simulink model "HDVPSG_DelayComp_NewRef_RealDrop_case1"  (R2019b)
settings: Solver=FixedStepDiscrete  StartTime=0.0  StopTime=28  FixedStep=UT.Ts_Veh  RelTol=1e-3
PostLoadFcn:
  | if any(exist('dsrtsu_mdlpostloadfcn', 'file') ~= 0), dsrtsu_mdlpostloadfcn('Execute', bdroot); end
InitFcn:
  | , if any(exist('dsmpb_private', 'file') ~= 0), dsmpb_private('dsmpb_mdlclblib', 'Init', bdroot); end,
values from neighbouring files (symbols this model uses):
  BETA_HDV_Leader = 50    [HDVPSG_DelayComp_NewRef_RealDrop_script_case1.m]
  BETA_PSG_Follower = 150    [HDVPSG_DelayComp_NewRef_RealDrop_script_case1.m]
  CtrlZone_Length = 250    [HDVPSG_DelayComp_NewRef_RealDrop_script_case1.m]
  DELTA_D_MIN = 5    [HDVPSG_DelayComp_NewRef_RealDrop_script_case1.m]
  DELTA_DR_MG_TCC = 15    [HDVPSG_DelayComp_NewRef_RealDrop_script_case1.m]
  HDV_AMAX = 1.3    [HDVPSG_DelayComp_NewRef_RealDrop_script_case1.m]
  HDV_AMIN = -2.5    [HDVPSG_DelayComp_NewRef_RealDrop_script_case1.m]
  HDV_first_v0 = 13    [HDVPSG_DelayComp_NewRef_RealDrop_script_case1.m]
  HDV_HighMu_D = 9    [HDVPSG_DelayComp_NewRef_RealDrop_script_case1.m]
  HDV_HighMu_I = 27    [HDVPSG_DelayComp_NewRef_RealDrop_script_case1.m]
  HDV_HighMu_P = 27    [HDVPSG_DelayComp_NewRef_RealDrop_script_case1.m]
  HDV_HighMu_TRFC = 0.7    [HDVPSG_DelayComp_NewRef_RealDrop_script_case1.m]
  HDV_last_v0 = 13    [HDVPSG_DelayComp_NewRef_RealDrop_script_case1.m]
  HDV_LowMu_D = 6    [HDVPSG_DelayComp_NewRef_RealDrop_script_case1.m]
  HDV_LowMu_I = 8    [HDVPSG_DelayComp_NewRef_RealDrop_script_case1.m]
  HDV_LowMu_P = 12    [HDVPSG_DelayComp_NewRef_RealDrop_script_case1.m]
  HDV_LowMu_TRFC = 0.6    [HDVPSG_DelayComp_NewRef_RealDrop_script_case1.m]
  Np_MPC = 20    [HDVPSG_DelayComp_NewRef_RealDrop_script_case1.m]
  PSG_AMAX = 3.2    [HDVPSG_DelayComp_NewRef_RealDrop_script_case1.m]
  PSG_AMIN = -6    [HDVPSG_DelayComp_NewRef_RealDrop_script_case1.m]
  PSG_end_v0 = 13    [HDVPSG_DelayComp_NewRef_RealDrop_script_case1.m]
  PSG_first_v0 = 13    [HDVPSG_DelayComp_NewRef_RealDrop_script_case1.m]
  PSG_HighMu_D = 15    [HDVPSG_DelayComp_NewRef_RealDrop_script_case1.m]
  PSG_HighMu_I = 125    [HDVPSG_DelayComp_NewRef_RealDrop_script_case1.m]
  PSG_HighMu_P = 75    [HDVPSG_DelayComp_NewRef_RealDrop_script_case1.m]
  PSG_HighMu_TRFC = 0.8    [HDVPSG_DelayComp_NewRef_RealDrop_script_case1.m]
  PSG_LowMu_D = 12    [HDVPSG_DelayComp_NewRef_RealDrop_script_case1.m]
  PSG_LowMu_I = 64    [HDVPSG_DelayComp_NewRef_RealDrop_script_case1.m]
  PSG_LowMu_P = 48    [HDVPSG_DelayComp_NewRef_RealDrop_script_case1.m]
  PSG_LowMu_TRFC = 0.7    [HDVPSG_DelayComp_NewRef_RealDrop_script_case1.m]
  PSG_middle_v0 = 13    [HDVPSG_DelayComp_NewRef_RealDrop_script_case1.m]
  Q_Leader = 1    [HDVPSG_DelayComp_NewRef_RealDrop_script_case1.m]
  Qd_dot_PSG_Follower = 2    [HDVPSG_DelayComp_NewRef_RealDrop_script_case1.m]
  Qd_PSG_Follower = 10    [HDVPSG_DelayComp_NewRef_RealDrop_script_case1.m]
  R_Leader = 20    [HDVPSG_DelayComp_NewRef_RealDrop_script_case1.m]
  R_PSG_Follower = 1    [HDVPSG_DelayComp_NewRef_RealDrop_script_case1.m]
  Recved_40_1 = Recved_Flag_Combined(47740,:)    [HDVPSG_DelayComp_NewRef_RealDrop_script_case1.m]
  Recved_40_2 = Recved_Flag_Combined(47780,:)    [HDVPSG_DelayComp_NewRef_RealDrop_script_case1.m]
  Recved_40_3 = Recved_Flag_Combined(49536,:)    [HDVPSG_DelayComp_NewRef_RealDrop_script_case1.m]
  Recved_40_4 = Recved_Flag_Combined(118106,:)    [HDVPSG_DelayComp_NewRef_RealDrop_script_case1.m]
  Rho_deltad_PSG_Follower = 1e3    (= 1000)    [HDVPSG_DelayComp_NewRef_RealDrop_script_case1.m]
  Rho_v_PSG_Follower = 1e3    (= 1000)    [HDVPSG_DelayComp_NewRef_RealDrop_script_case1.m]
  T_ADE = 0.01    [HDVPSG_DelayComp_NewRef_RealDrop_script_case1.m]
  V_MAX = 40    [HDVPSG_DelayComp_NewRef_RealDrop_script_case1.m]
  V_MIN = 0    [HDVPSG_DelayComp_NewRef_RealDrop_script_case1.m]
  VR_MG_TCC = 15    [HDVPSG_DelayComp_NewRef_RealDrop_script_case1.m]
undefined symbols (not defined in the file or in its folder): DiscIntNeverNeededParam, UT
libraries: simulink x46
(part 3 of 16)

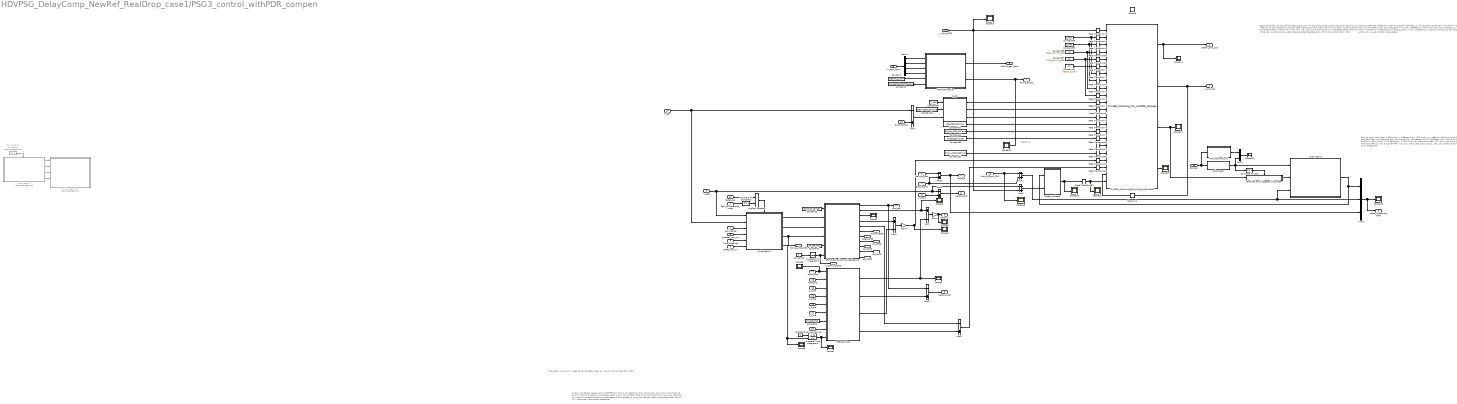
== system HDVPSG_DelayComp_NewRef_RealDrop_case1/PSG3_control_withPDR_compen ==
  note: As the immediate leader cannot PERFECTLY follow its reference, then there may be minor initial tracking errors in terms of delta_d and delta_d_dot, which can trigger large initial command
      |
      | One way to overcome this issue is to recalculate the parameters of the leader by using the leader's real-time states data. But it will introduce inconsistant reference
  note: For the case when Recv's frequency is different from MPC, then you need to make sure that the predicted step matches the real world time. So, we create a novel Lost-step block
      |
      | The commented one only works when V2VC freqeucny = MPC
      |
      | The max prediction step is 21, so if you have Large Sampling Period with a higher PDR, you may have step lost over 21. We just use the last one to fulfill the others.
  note: Adaptive
  note: Because Hc =1, so the diff of delta_d_dot_pre will equal the delta_ddot_hat as the MPC input.
      | That means, we cannot get the next Np step delta_ddot from MPC's solution; so the a of front car needs to be estimated in other ways.
      | For now, we just hold a_front once it is lost
      |
      | Because of a_front's influence, we cannot have accurate predicted delta_d_dot within the horizon from MPC
  note: Use the predicted states from MPC to replace lost delta_d, the results is quitewell;
      |
      | However, it does not work for delta_d_dot, the prediciton of d_dot is affected by both your command (delta_v_r), but more importantly, it depends on delta_d_ddot, which is affected by a_front. Unless you can predict a_front, or you cannot do it accurately.
  note: The green inputs only need to be inputted once. So, we do not consider their PDR.
  Ego_CtrL_enabled_Index : Inport
  t_all_leader : Inport  Port=2
  t_leader_has_run : Inport  Port=3
  t_PRE_has_run : Inport  Port=4
  Time_headway : Inport  Port=5
  Front_to_end : Inport  Port=6
  Ego_to_end : Inport  Port=7
  v_Front : Inport  Port=8
  v_Ego : Inport  Port=9
  a_Ego : Inport  Port=10
  XY_ego_front : Inport  Port=11
  Reset_sig : Inport  Port=12
  Front_to_end_PDR : Inport  Port=13
  v_Front_PDR : Inport  Port=14
  a_Front_PDR : Inport  Port=15
  Recved : Inport  Port=16
  alpha_pre : Inport  Port=17
  beta_pre : Inport  Port=18
  c_1_pre : Inport  Port=19
  c_2_pre : Inport  Port=20
  c_3_pre : Inport  Port=21
  c_4_pre : Inport  Port=22
  T_all_to_MP_pre : Inport  Port=23
  Enable : EnablePort
  Add : Sum  Inputs=+-
  Add{1..3,5..8} (7 alike) : Sum  Inputs=-+
  Add4 : Sum  Inputs=+-
  CVXGEN_Following_Car_Dist_Ctrl_NonSoft2 : S-Function  Description=Simulink:masks:SFunctionBuilder_MD  InitFcn=try, set_param(gcb,'FunctionName','CVXGEN_Following_Car_withPDR_Compen'), end  FunctionName=CVXGEN_Following_Car_withPDR_Compen  SFunctionModules=CVXGEN_Following_Car_withPDR_Compen_wrapper solver util matrix_support ldl  SFunctionDeploymentMode=off  EnableBusSupport=off
      mask init: same as HDVPSG_DelayComp_NewRef_RealDrop_case1/HDV2_control_withPDR_compen/CVXGEN_Following_Car_Dist_Ctrl_NonSoft2
      settings: CopyFcn=set_param(gcbh,'LinkStatus','none')  PreSaveFcn=try, set_param(gcb,'FunctionName','CVXGEN_Following_Car_withPDR_Compen'), end  OpenFcn=sfunctionwizard(gcbh)
      mask Display: plot(val(:,1),val(:,2)),disp(sys), port_label('input',1,'v_front_car'), port_label('input',2,'vmax'), port_label('input',3,'vmin'), port_label('input',4,'deltav_max'), port_label('input',5,'deltav_min'), port_label('input',6,'deltad_min'), port_label('input',7,'vcmd_max'), port_label('input',8,'vcmd_min'), port_label('input',9,'delta_vcmd_max'), port_label('input',10,'delta_vcmd_min'), port_label('input',11,'A'), port_label('input',12,'B'), port_label('input',13,'d_k'), port_label('input',14,'Q_deltad'), port_label('input',15,'Q_deltad_dot'), port_label('input',16,'R'), port_label('input',17,'Rho_deltad'), port_label('input',18,'Rho_v'), port_label('input',19,'deltad_r'), port_label('input',20,'deltad_dot_r'), port_label('input',21,'v_cmd_last'), port_label('input',22,'x_0'), port_label('output',1,'delta_v_cmd_opt'), port_label('output',2,'v_cmd_opt'), port_label('output',3,'delta_d_pre'), port_label('output',4,'delta_d_dot_pre')
  Compare To Constant2 : simulink/Logic and Bit Operations/Compare To Constant  relop===  const=1  OutDataTypeStr=boolean
  Compare To Constant3 : simulink/Logic and Bit Operations/Compare To Constant  Commented=on  relop===  const=1  OutDataTypeStr=boolean
  Compare To Zero : simulink/Logic and Bit Operations/Compare To Zero  relop===  OutDataTypeStr=boolean
  Constant : Constant  Value=DELTA_D_MIN
  Constant2 : Constant  Value=Rho_deltad_PSG_Follower
  Constant3 : Constant
  Constant4 : Constant  Value=VR_MG_TCC
  Constant42 : Constant  Value=T_ADE
  Constant43 : Constant  Value=Qd_PSG_Follower
  Constant44 : Constant  Value=Qd_dot_PSG_Follower
  Constant45 : Constant  Value=DELTA_D_MIN
  Constant5 : Constant
  Constant50 : Constant  Value=R_PSG_Follower
  Constant51 : Constant  Value=Rho_v_PSG_Follower
  Constant55 : Constant  Value=PSG_AMAX*T_ADE
  Constant57 : Constant  Value=PSG_AMIN*T_ADE
  Constant58 : Constant  Value=V_MAX
  Constant59 : Constant  Value=V_MIN
  Constant6 : Constant  Value=CtrlZone_Length
  Constant61 : Constant  Value=BETA_PSG_Follower
  Constant7 : Constant  Value=VR_MG_TCC
  Demux : Demux
  Discrete-Time Integrator1 : DiscreteIntegrator  SampleTime=-1  ICPrevOutput=DiscIntNeverNeededParam  ICPrevScaledInput=DiscIntNeverNeededParam
  Discrete-Time Integrator2 : DiscreteIntegrator  InitialConditionSource=external  SampleTime=-1  ICPrevOutput=DiscIntNeverNeededParam  ICPrevScaledInput=DiscIntNeverNeededParam
  Enabled and Triggered Subsystem : Subsystem  TreatAsAtomicUnit=on
  Gain1 : Gain  Gain=-1
  Gain4 : Gain  Gain=-1
  Logical Operator : Logic  Operator=OR  AllPortsSameDT=off  OutDataTypeStr=boolean
  MATLAB Function : MATLAB Function  TreatAsAtomicUnit=on
  MATLAB Function2 : MATLAB Function  TreatAsAtomicUnit=on
  Memory2 : Memory  InitialCondition=PSG_end_v0
  Mux2 : Mux  Inputs=3
  Mux3 : Mux  Inputs=2
  PRE_OPT_Pos : MATLAB Function  TreatAsAtomicUnit=on
  Rate Transition{6,48..50,68,70..85} (21 alike) : RateTransition
  SELF_Optimal_Control_Reference : MATLAB Function  TreatAsAtomicUnit=on
  Scope{1..8,10..12,14..19,21} (18 alike) : Scope
  States_update2 : MATLAB Function  TreatAsAtomicUnit=on
  Subsystem : Subsystem
  Subsystem17 : Subsystem  Commented=on
  Subsystem18 : Subsystem  Commented=on
  Subsystem2 : Subsystem
  Subsystem3 : Subsystem
  Sys3 : MATLAB Function  TreatAsAtomicUnit=on
  v_cmd_opt : Outport
  deltav_cmd_opt : Outport  Port=2
  delta_dr : Outport  Port=3
  delta_d : Outport  Port=4
  delta_dr_dot : Outport  Port=5
  delta_d_dot : Outport  Port=6
  Rho_d_adapt : Outport  Port=7
  AbsDis_ego_front : Outport  Port=8
  delta_d_against_PDR : Outport  Port=9
  opt_spd : Outport  Port=10
  alpha_PSG3 : Outport  Port=11
  beta_PSG3 : Outport  Port=12
  c1_PSG3 : Outport  Port=13
  c2_PSG3 : Outport  Port=14
  c3_PSG3 : Outport  Port=15
  c4_PSG3 : Outport  Port=16
  Tall_to_MP_PSG3 : Outport  Port=17
  t_hasrun_PSG3 : Outport  Port=18
  wires:
  SELF_Optimal_Control_Reference/11(c_4) -> c4_PSG3/1
  SELF_Optimal_Control_Reference/10(c_3) -> c3_PSG3/1
  SELF_Optimal_Control_Reference/9(c_2) -> c2_PSG3/1
  SELF_Optimal_Control_Reference/8(c_1) -> c1_PSG3/1
  SELF_Optimal_Control_Reference/7(beta) -> beta_PSG3/1
  SELF_Optimal_Control_Reference/6(alpha) -> alpha_PSG3/1
  SELF_Optimal_Control_Reference/3(opt_acc) -> Scope1/1
  Gain4/1 -> Scope4/1, Rate Transition84/1
  Gain1/1 -> Scope5/1, delta_dr/1
  Add5/1 -> Rate Transition85/1
  SELF_Optimal_Control_Reference/5(opt_spd_vec) -> Add5/1
  PRE_OPT_Pos/4(opt_spd_pre_vec) -> Add5/2
  PRE_OPT_Pos/3(opt_pos_pre_vec) -> Add4/2
  SELF_Optimal_Control_Reference/4(opt_pos_vec) -> Add4/1
  Add4/1 -> Gain4/1
  Add3/1 -> delta_dr_dot/1
  PRE_OPT_Pos/2(opt_spd_pre) -> Add3/2
  Add/1 -> Gain1/1
  PRE_OPT_Pos/1(opt_pos_pre) -> Scope2/1, Add/2
  T_all_to_MP_pre/1 -> PRE_OPT_Pos/8(T_all_to_MP_pre)
  Subsystem3/4(t_PRE_has_run_ini) -> Scope8/1, Discrete-Time Integrator2/2
  t_PRE_has_run/1 -> Subsystem3/6(t_PRE_has_run)
  Constant5/1 -> Discrete-Time Integrator2/1
  Discrete-Time Integrator2/1 -> Scope7/1, PRE_OPT_Pos/9(t_aft_trigger_pre)
  Constant4/1 -> PRE_OPT_Pos/7(v_mp)
  c_4_pre/1 -> PRE_OPT_Pos/6(c_4_pre)
  c_3_pre/1 -> PRE_OPT_Pos/5(c_3_pre)
  c_2_pre/1 -> PRE_OPT_Pos/4(c_2_pre)
  c_1_pre/1 -> PRE_OPT_Pos/3(c_1_pre)
  beta_pre/1 -> PRE_OPT_Pos/2(beta_pre)
  alpha_pre/1 -> Scope6/1, PRE_OPT_Pos/1(alpha_pre)
  SELF_Optimal_Control_Reference/2(opt_pos) -> Scope3/1, Add/1
  SELF_Optimal_Control_Reference/1(opt_spd) -> opt_spd/1, Add3/1
  Subsystem3/3(T_all_to_MP_ego) -> Tall_to_MP_PSG3/1, SELF_Optimal_Control_Reference/4(T_all_to_MP)
  Subsystem3/2(a_ego_ini) -> SELF_Optimal_Control_Reference/3(a_ini)
  Subsystem3/1(v_ego_ini) -> SELF_Optimal_Control_Reference/2(v_ini)
  Constant6/1 -> SELF_Optimal_Control_Reference/1(L_ctz)
  Constant7/1 -> SELF_Optimal_Control_Reference/5(v_mp)
  Discrete-Time Integrator1/1 -> SELF_Optimal_Control_Reference/6(t_aft_trigger), t_hasrun_PSG3/1
  Constant3/1 -> Discrete-Time Integrator1/1
  Subsystem/1(Lost_Step) -> Subsystem2/1(Lost_Step), Compare To Zero/1, Mux3/2
  Mux3/1 -> Scope21/1
  MATLAB Function2/1(Lost_Step) -> Mux3/1
  a_Front_PDR/1 -> Add7/2
  v_Front_PDR/1 -> Scope17/1, Rate Transition74/1, Add2/2
  Front_to_end_PDR/1 -> Scope19/1, Add1/1
  Add1/1 -> Subsystem2/3(delta_d_measure), Mux2/2
  Reset_sig/1 -> Logical Operator/1
  Logical Operator/1 -> Subsystem3/Enable
  Compare To Constant2/1 -> Logical Operator/2
  t_leader_has_run/1 -> Subsystem3/4(t_leader_has_run)
  Time_headway/1 -> Subsystem3/5(Time_headway)
  Constant57/1 -> Rate Transition70/1, Rate Transition68/1
  Rate Transition73/1 -> CVXGEN_Following_Car_Dist_Ctrl_NonSoft2/13
  Rate Transition83/1 -> CVXGEN_Following_Car_Dist_Ctrl_NonSoft2/22, Scope12/1
  a_Ego/1 -> Add7/1, Subsystem3/2(a_ego)  "a_ego"
  Ego_to_end/1 -> Add1/2, Add8/2
  Constant51/1 -> Rate Transition82/1
  Rate Transition68/1 -> CVXGEN_Following_Car_Dist_Ctrl_NonSoft2/5
  Rate Transition70/1 -> CVXGEN_Following_Car_Dist_Ctrl_NonSoft2/10
  Constant59/1 -> Rate Transition77/1, Rate Transition49/1
  CVXGEN_Following_Car_Dist_Ctrl_NonSoft2/1 -> deltav_cmd_opt/1, Scope11/1
  v_Front/1 -> Add6/2
  Rate Transition79/1 -> CVXGEN_Following_Car_Dist_Ctrl_NonSoft2/15
  v_Ego/1 -> Subsystem3/1(v_ego), Add6/1, Add2/1
  Constant58/1 -> Rate Transition76/1, Rate Transition48/1
  Rate Transition77/1 -> CVXGEN_Following_Car_Dist_Ctrl_NonSoft2/8
  Constant55/1 -> Rate Transition78/1, Rate Transition50/1
  Constant44/1 -> Rate Transition79/1
  Constant42/1 -> Sys3/1(Ts)
  Sys3/3(dk) -> Rate Transition73/1
  Rate Transition84/1 -> CVXGEN_Following_Car_Dist_Ctrl_NonSoft2/19
  Rate Transition71/1 -> CVXGEN_Following_Car_Dist_Ctrl_NonSoft2/11
  Rate Transition82/1 -> CVXGEN_Following_Car_Dist_Ctrl_NonSoft2/18
  Constant43/1 -> Rate Transition75/1
  Constant50/1 -> Rate Transition80/1
  CVXGEN_Following_Car_Dist_Ctrl_NonSoft2/2 -> v_cmd_opt/1, Memory2/1  "v_cmd_opt"
  Rate Transition81/1 -> CVXGEN_Following_Car_Dist_Ctrl_NonSoft2/17
  Constant61/1 -> Sys3/2(beta)
  MATLAB Function/2(Rho_delta_d_adpt) -> Rho_d_adapt/1, Scope10/1
  Rate Transition85/1 -> CVXGEN_Following_Car_Dist_Ctrl_NonSoft2/20
  Rate Transition49/1 -> CVXGEN_Following_Car_Dist_Ctrl_NonSoft2/3
  Sys3/2(B) -> Rate Transition6/1
  Rate Transition6/1 -> CVXGEN_Following_Car_Dist_Ctrl_NonSoft2/12
  Memory2/1 -> CVXGEN_Following_Car_Dist_Ctrl_NonSoft2/21
  Add8/1 -> Mux2/3, delta_d/1
  Rate Transition74/1 -> CVXGEN_Following_Car_Dist_Ctrl_NonSoft2/1
  Add7/1 -> Sys3/3(delta_d_ddot_hat)
  Ego_CtrL_enabled_Index/1 -> Compare To Constant2/1
  Rate Transition48/1 -> CVXGEN_Following_Car_Dist_Ctrl_NonSoft2/2
  Sys3/1(A) -> Rate Transition71/1
  Constant45/1 -> Rate Transition72/1
  Rate Transition80/1 -> CVXGEN_Following_Car_Dist_Ctrl_NonSoft2/16
  States_update2/1(x0) -> Scope16/1, Rate Transition83/1
  Rate Transition50/1 -> CVXGEN_Following_Car_Dist_Ctrl_NonSoft2/4
  Rate Transition78/1 -> CVXGEN_Following_Car_Dist_Ctrl_NonSoft2/9
  Rate Transition76/1 -> CVXGEN_Following_Car_Dist_Ctrl_NonSoft2/7
  Rate Transition75/1 -> CVXGEN_Following_Car_Dist_Ctrl_NonSoft2/14
  Rate Transition72/1 -> CVXGEN_Following_Car_Dist_Ctrl_NonSoft2/6
  Add6/1 -> delta_d_dot/1
  t_all_leader/1 -> Subsystem3/3(t_all_leader)
  XY_ego_front/1 -> Demux/1
  Demux/1 -> MATLAB Function/1(X_Ego)  "X_ego"
  Demux/2 -> MATLAB Function/2(Y_Ego)  "Y_ego"
  Demux/3 -> MATLAB Function/3(X_Front)  "X_front"
  Demux/4 -> MATLAB Function/4(Y_Front)  "Y_front"
  Constant/1 -> MATLAB Function/5(DELTA_D_MIN)
  Constant2/1 -> MATLAB Function/6(Rho_delta_dMAX)
  Subsystem17/1(a_0) -> Subsystem18/1(a0)
  Subsystem17/3(a_2) -> Subsystem18/3(a2)
  Subsystem17/4(a_3) -> Subsystem18/4(a3)
  Subsystem17/2(a_1) -> Subsystem18/2(a1)
  Compare To Constant3/1 -> Subsystem17/Enable
  MATLAB Function/1(REALWORLD_DIST) -> AbsDis_ego_front/1
  Recved/1 -> MATLAB Function2/1(Recv), Subsystem/1(Recv)
  CVXGEN_Following_Car_Dist_Ctrl_NonSoft2/3 -> Scope14/1, Enabled and Triggered Subsystem/1(delta_d_pre)
  CVXGEN_Following_Car_Dist_Ctrl_NonSoft2/4 -> Scope15/1
  Compare To Zero/1 -> Enabled and Triggered Subsystem/Enable
  Enabled and Triggered Subsystem/1(delta_d_pre_freeze) -> Subsystem2/2(delta_d_pre_freeze_if_lost)
  Subsystem2/1(delta_d_enhanced) -> States_update2/1(delta_d), Mux2/1
  Mux2/1 -> delta_d_against_PDR/1, Scope18/1
  Front_to_end/1 -> Add8/1
  Add2/1 -> States_update2/2(delta_d_dot)

== system HDVPSG_DelayComp_NewRef_RealDrop_case1/Subsystem1 ==
  vxr_PSG_middle : Inport
  Dist_to_MP : Inport  Port=2
  Constant56 : Constant  Value=PSG_middle_v0
  PSG_first : Subsystem
  Subsystem4 : Subsystem
  Subsystem5 : Subsystem
  Subsystem6 : Subsystem
  Subsystem7 : Subsystem
  vx_PSG_middle : Outport
  HighMu : Outport  Port=2
  wires:
  Dist_to_MP/1 -> Subsystem7/1(Dist_to_MP), Subsystem6/1(Dist_to_MP), Subsystem5/1(Dist_to_MP), Subsystem4/1(Dist_to_MP)
  PSG_first/1(vx) -> vx_PSG_middle/1
  Subsystem7/1(PSG_Mu) -> PSG_first/5(TRFC)
  Subsystem6/1(PSG_D) -> PSG_first/4(PID_D)
  Subsystem5/1(PSG_I) -> PSG_first/3(PID_I)
  Subsystem4/1(PSG_P) -> PSG_first/2(PID_P)
  Constant56/1 -> PSG_first/6(v_ini)
  vxr_PSG_middle/1 -> PSG_first/1(vxr)
  Subsystem4/2(HighMu) -> HighMu/1

== system HDVPSG_DelayComp_NewRef_RealDrop_case1/Subsystem10 ==
  dis_to_MP : Inport
  Add5 : Sum
  Compare To Constant1 : simulink/Logic and Bit Operations/Compare To Constant  relop=<=  const=CtrlZone_Length  OutDataTypeStr=boolean
  Compare To Constant2 : simulink/Logic and Bit Operations/Compare To Constant  relop=>  const=0  OutDataTypeStr=boolean
  Data Type Conversion : DataTypeConversion
  Delay : Delay  DelayLength=1
  Ctrl_enabled : Outport
  Ctrl_enable_Index : Outport  Port=2
  wires:
  dis_to_MP/1 -> Compare To Constant1/1
  Compare To Constant1/1 -> Data Type Conversion/1
  Compare To Constant2/1 -> Ctrl_enabled/1
  Add5/1 -> Delay/1
  Delay/1 -> Compare To Constant2/1, Add5/2, Ctrl_enable_Index/1
  Data Type Conversion/1 -> Add5/1

== system HDVPSG_DelayComp_NewRef_RealDrop_case1/Subsystem11 ==
  dis_to_MP : Inport
  Add5 : Sum
  Compare To Constant1 : simulink/Logic and Bit Operations/Compare To Constant  relop=<=  const=CtrlZone_Length  OutDataTypeStr=boolean
  Compare To Constant2 : simulink/Logic and Bit Operations/Compare To Constant  relop=>  const=0  OutDataTypeStr=boolean
  Data Type Conversion : DataTypeConversion
  Delay : Delay  DelayLength=1
  Ctrl_enabled : Outport
  Ctrl_enable_Index : Outport  Port=2
  wires:
  Data Type Conversion/1 -> Add5/1
  Delay/1 -> Ctrl_enable_Index/1, Add5/2, Compare To Constant2/1
  Add5/1 -> Delay/1
  Compare To Constant2/1 -> Ctrl_enabled/1
  Compare To Constant1/1 -> Data Type Conversion/1
  dis_to_MP/1 -> Compare To Constant1/1

== system HDVPSG_DelayComp_NewRef_RealDrop_case1/Subsystem12 ==
  note: With a_dot, the packet drop estimation can become, worse
  note: Unfortunately,
      | Solution a. Remain till updated and
      | Solution b. Linear extrapolation with a_dot = 0
      |
      | b's inprovement is just marginal
  d2MP_PDR : Inport
  v_PDR : Inport  Port=2
  a_PDR : Inport  Port=3
  Recved : Inport  Port=4
  lost_period : Inport  Port=5
  ARE_First_Order_Derivative_[1,0,0]5 : Subsystem  TreatAsAtomicUnit=on
  Add1 : Sum
  Add2 : Sum  Inputs=3
  Add3 : Sum  Inputs=4
  Fcn : Fcn  Expr=u^2/2
  Fcn1 : Fcn  Expr=u^2/2
  Fcn2 : Fcn  Expr=u^3/6
  Filter_Ts5 : DiscretePulseGenerator  PulseType=Time based  Period=T_ADE*2  PulseWidth=50
  Gain : Gain  Gain=-1
  Gain1 : Gain  Gain=-1
  Gain2 : Gain  Gain=-1
  Gain3 : Gain  Gain=0
  Memory1 : Memory
  Memory2 : Memory
  Memory3 : Memory
  Product{1..6} (6 alike) : Product
  Switch1 : Switch  Criteria=u2 > Threshold
  Switch2 : Switch  Criteria=u2 > Threshold
  Switch3 : Switch  Criteria=u2 > Threshold
  lost_period1 : InportShadow  Port=5
  lost_period2 : InportShadow  Port=5
  d2MP_PDR_enhanced_by_Inertia_Integral : Outport
  v_PDR_enhanced_by_Inertia_Integral : Outport  Port=2
  a_PDR_enhanced_by_Inertia_Integral : Outport  Port=3
  wires:
  ARE_First_Order_Derivative_[1,0,0]5/1(a_dot_hat) -> Gain3/1
  Switch1/1 -> ARE_First_Order_Derivative_[1,0,0]5/1(a), Add1/2, a_PDR_enhanced_by_Inertia_Integral/1, Product2/1, Product5/1
  a_PDR/1 -> Switch1/1
  Product1/1 -> Add1/1
  lost_period/1 -> Product1/2
  Memory1/1 -> Switch1/3
  Add1/1 -> Memory1/1
  Recved/1 -> Switch1/2, Switch3/2, Switch2/2
  Filter_Ts5/1 -> ARE_First_Order_Derivative_[1,0,0]5/Trigger
  v_PDR/1 -> Switch2/1
  lost_period1/1 -> Fcn/1, Product2/2
  Product2/1 -> Add2/2
  Add2/1 -> Memory2/1
  Product3/1 -> Add2/3
  Fcn/1 -> Product3/1
  Memory2/1 -> Switch2/3
  Switch2/1 -> Add2/1, v_PDR_enhanced_by_Inertia_Integral/1, Product4/1
  d2MP_PDR/1 -> Switch3/1
  Memory3/1 -> Switch3/3
  Add3/1 -> Memory3/1
  Switch3/1 -> Add3/1, d2MP_PDR_enhanced_by_Inertia_Integral/1
  Product4/1 -> Gain/1
  lost_period2/1 -> Product4/2, Fcn1/1, Fcn2/1
  Gain/1 -> Add3/2
  Product5/1 -> Gain1/1
  Gain1/1 -> Add3/3
  Fcn1/1 -> Product5/2
  Gain2/1 -> Add3/4
  Product6/1 -> Gain2/1
  Fcn2/1 -> Product6/2
  Gain3/1 -> Product6/1, Product3/2, Product1/1

== system HDVPSG_DelayComp_NewRef_RealDrop_case1/Subsystem13 ==
  dis_to_MP : Inport
  Add5 : Sum
  Compare To Constant1 : simulink/Logic and Bit Operations/Compare To Constant  relop=<=  const=CtrlZone_Length  OutDataTypeStr=boolean
  Compare To Constant2 : simulink/Logic and Bit Operations/Compare To Constant  relop=>  const=0  OutDataTypeStr=boolean
  Data Type Conversion : DataTypeConversion
  Delay : Delay  DelayLength=1
  Ctrl_enabled : Outport
  Ctrl_enable_Index : Outport  Port=2
  wires:
  Data Type Conversion/1 -> Add5/1
  Delay/1 -> Ctrl_enable_Index/1, Add5/2, Compare To Constant2/1
  Add5/1 -> Delay/1
  Compare To Constant2/1 -> Ctrl_enabled/1
  Compare To Constant1/1 -> Data Type Conversion/1
  dis_to_MP/1 -> Compare To Constant1/1

== system HDVPSG_DelayComp_NewRef_RealDrop_case1/Subsystem15 ==
  note: We assume you know if a packet is lost or not.
  Front_to_end : Inport
  v_Front : Inport  Port=2
  a_Front : Inport  Port=3
  Add : Sum
  Constant : Constant
  Data Type Conversion2 : DataTypeConversion
  Enabled Subsystem1 : Subsystem  TreatAsAtomicUnit=on
  Enabled Subsystem2 : Subsystem  TreatAsAtomicUnit=on
  Enabled Subsystem3 : Subsystem  TreatAsAtomicUnit=on
  Memory : Memory
  Mux : Mux  Inputs=2
  Mux1 : Mux  Inputs=2
  Mux2 : Mux  Inputs=2
  Recved_40%_4 : Lookup_n-D  NumberOfTableDimensions=1  BreakpointsForDimension1=1:3000  Table=Recved_40_4  InternalRulePriority=Speed  RndMeth=Simplest  InputSameDT=on
  Scope{,1..2,4} (4 alike) : Scope
  Front_to_end_PDR : Outport
  v_Front_PDR : Outport  Port=2
  a_Front_PDR : Outport  Port=3
  Recved : Outport  Port=4
  wires:
  Data Type Conversion2/1 -> Scope4/1, Recved/1
  Mux2/1 -> Scope2/1
  Enabled Subsystem2/1(v_Front_PDR) -> v_Front_PDR/1, Mux1/1
  v_Front/1 -> Enabled Subsystem2/1(v_Front), Mux1/2
  Mux1/1 -> Scope1/1
  Mux/1 -> Scope/1
  Front_to_end/1 -> Enabled Subsystem1/1(Front_to_end), Mux/2
  a_Front/1 -> Enabled Subsystem3/1(a_Front), Mux2/2
  Enabled Subsystem3/1(a_Front_PDR) -> a_Front_PDR/1, Mux2/1
  Enabled Subsystem1/1(Front_to_end_PDR) -> Front_to_end_PDR/1, Mux/1
  Memory/1 -> Recved_40%_4/1, Add/2  "Index_Step"
  Add/1 -> Memory/1
  Constant/1 -> Add/1
  Recved_40%_4/1 -> Enabled Subsystem1/Enable, Data Type Conversion2/1, Enabled Subsystem3/Enable, Enabled Subsystem2/Enable

== system HDVPSG_DelayComp_NewRef_RealDrop_case1/Subsystem2 ==
  vxr_PSG_end : Inport
  Dist_to_MP : Inport  Port=2
  Constant56 : Constant  Value=PSG_end_v0
  PSG_first : Subsystem
  Subsystem4 : Subsystem
  Subsystem5 : Subsystem
  Subsystem6 : Subsystem
  Subsystem7 : Subsystem
  vx_PSG_end : Outport
  HighMu : Outport  Port=2
  wires:
  vxr_PSG_end/1 -> PSG_first/1(vxr)
  Constant56/1 -> PSG_first/6(v_ini)
  Subsystem4/1(PSG_P) -> PSG_first/2(PID_P)
  Subsystem5/1(PSG_I) -> PSG_first/3(PID_I)
  Subsystem6/1(PSG_D) -> PSG_first/4(PID_D)
  Subsystem7/1(PSG_Mu) -> PSG_first/5(TRFC)
  PSG_first/1(vx) -> vx_PSG_end/1
  Dist_to_MP/1 -> Subsystem4/1(Dist_to_MP), Subsystem5/1(Dist_to_MP), Subsystem6/1(Dist_to_MP), Subsystem7/1(Dist_to_MP)
  Subsystem4/2(HighMu) -> HighMu/1

== system HDVPSG_DelayComp_NewRef_RealDrop_case1/Subsystem29 ==
  vxr_PSG_first : Inport
  Dist_to_MP : Inport  Port=2
  Constant56 : Constant  Value=PSG_first_v0
  PSG_first : Subsystem
  Subsystem4 : Subsystem
  Subsystem5 : Subsystem
  Subsystem6 : Subsystem
  Subsystem7 : Subsystem
  vx_PSG_first : Outport
  HighMu : Outport  Port=2
  wires:
  vxr_PSG_first/1 -> PSG_first/1(vxr)
  Constant56/1 -> PSG_first/6(v_ini)
  Subsystem4/1(PSG_P) -> PSG_first/2(PID_P)
  Subsystem5/1(PSG_I) -> PSG_first/3(PID_I)
  Subsystem6/1(PSG_D) -> PSG_first/4(PID_D)
  Subsystem7/1(PSG_Mu) -> PSG_first/5(TRFC)
  PSG_first/1(vx) -> vx_PSG_first/1
  Dist_to_MP/1 -> Subsystem4/1(Dist_to_MP), Subsystem5/1(Dist_to_MP), Subsystem6/1(Dist_to_MP), Subsystem7/1(Dist_to_MP)
  Subsystem4/2(HighMu) -> HighMu/1

== system HDVPSG_DelayComp_NewRef_RealDrop_case1/Subsystem3 ==
  vxr_HDV_end : Inport
  Dist_to_MP : Inport  Port=2
  Constant52 : Constant  Value=HDV_last_v0
  HDV_first : Subsystem
  Subsystem16 : Subsystem
  Subsystem17 : Subsystem
  Subsystem18 : Subsystem
  Subsystem7 : Subsystem
  vx_HDV_end : Outport
  HighMu : Outport  Port=2
  wires:
  Dist_to_MP/1 -> Subsystem7/1(Dist_to_MP), Subsystem18/1(Dist_to_MP), Subsystem17/1(Dist_to_MP), Subsystem16/1(Dist_to_MP)
  HDV_first/1(vx) -> vx_HDV_end/1
  Subsystem17/1(HDV_I) -> HDV_first/3(PID_I)
  Constant52/1 -> HDV_first/6(v_ini)
  Subsystem7/1(HDV_Mu) -> HDV_first/5(TRFC)
  vxr_HDV_end/1 -> HDV_first/1(vxr)
  Subsystem16/1(HDV_P) -> HDV_first/2(PID_P)
  Subsystem18/1(HDV_D) -> HDV_first/4(PID_D)
  Subsystem16/2(HighMu) -> HighMu/1

== system HDVPSG_DelayComp_NewRef_RealDrop_case1/Subsystem4 ==
  note: We assume you know if a packet is lost or not.
  Front_to_end : Inport
  v_Front : Inport  Port=2
  a_Front : Inport  Port=3
  Add : Sum
  Constant : Constant
  Data Type Conversion2 : DataTypeConversion
  Enabled Subsystem1 : Subsystem  TreatAsAtomicUnit=on
  Enabled Subsystem2 : Subsystem  TreatAsAtomicUnit=on
  Enabled Subsystem3 : Subsystem  TreatAsAtomicUnit=on
  Memory : Memory
  Mux : Mux  Inputs=2
  Mux1 : Mux  Inputs=2
  Mux2 : Mux  Inputs=2
  Recved_40%_2 : Lookup_n-D  NumberOfTableDimensions=1  BreakpointsForDimension1=1:3000  Table=Recved_40_2  InternalRulePriority=Speed  RndMeth=Simplest  InputSameDT=on
  Scope{,1..2,4} (4 alike) : Scope
  Front_to_end_PDR : Outport
  v_Front_PDR : Outport  Port=2
  a_Front_PDR : Outport  Port=3
  Recved : Outport  Port=4
  wires:
  Data Type Conversion2/1 -> Scope4/1, Recved/1
  Mux2/1 -> Scope2/1
  Enabled Subsystem2/1(v_Front_PDR) -> v_Front_PDR/1, Mux1/1
  v_Front/1 -> Enabled Subsystem2/1(v_Front), Mux1/2
  Mux1/1 -> Scope1/1
  Mux/1 -> Scope/1
  Front_to_end/1 -> Enabled Subsystem1/1(Front_to_end), Mux/2
  a_Front/1 -> Enabled Subsystem3/1(a_Front), Mux2/2
  Enabled Subsystem3/1(a_Front_PDR) -> a_Front_PDR/1, Mux2/1
  Enabled Subsystem1/1(Front_to_end_PDR) -> Front_to_end_PDR/1, Mux/1
  Memory/1 -> Recved_40%_2/1, Add/2  "Index_Step"
  Add/1 -> Memory/1
  Constant/1 -> Add/1
  Recved_40%_2/1 -> Enabled Subsystem3/Enable, Enabled Subsystem2/Enable, Enabled Subsystem1/Enable, Data Type Conversion2/1

== system HDVPSG_DelayComp_NewRef_RealDrop_case1/Subsystem5 ==
  note: We assume you know if a packet is lost or not.
  Front_to_end : Inport
  v_Front : Inport  Port=2
  a_Front : Inport  Port=3
  Add : Sum
  Constant : Constant
  Data Type Conversion2 : DataTypeConversion
  Enabled Subsystem1 : Subsystem  TreatAsAtomicUnit=on
  Enabled Subsystem2 : Subsystem  TreatAsAtomicUnit=on
  Enabled Subsystem3 : Subsystem  TreatAsAtomicUnit=on
  Memory : Memory
  Mux : Mux  Inputs=2
  Mux1 : Mux  Inputs=2
  Mux2 : Mux  Inputs=2
  Recved_40%_1 : Lookup_n-D  NumberOfTableDimensions=1  BreakpointsForDimension1=1:3000  Table=Recved_40_1  InternalRulePriority=Speed  RndMeth=Simplest  InputSameDT=on
  Scope{,1..4} (5 alike) : Scope
  Front_to_end_PDR : Outport
  v_Front_PDR : Outport  Port=2
  a_Front_PDR : Outport  Port=3
  Recved : Outport  Port=4
  wires:
  Add/1 -> Memory/1
  Memory/1 -> Add/2, Recved_40%_1/1, Scope3/1  "Index_Step"
  Enabled Subsystem1/1(Front_to_end_PDR) -> Mux/1, Front_to_end_PDR/1
  Enabled Subsystem3/1(a_Front_PDR) -> Mux2/1, a_Front_PDR/1
  a_Front/1 -> Mux2/2, Enabled Subsystem3/1(a_Front)
  Front_to_end/1 -> Mux/2, Enabled Subsystem1/1(Front_to_end)
  Mux/1 -> Scope/1
  Mux1/1 -> Scope1/1
  v_Front/1 -> Mux1/2, Enabled Subsystem2/1(v_Front)
  Enabled Subsystem2/1(v_Front_PDR) -> Mux1/1, v_Front_PDR/1
  Mux2/1 -> Scope2/1
  Data Type Conversion2/1 -> Recved/1, Scope4/1
  Constant/1 -> Add/1
  Recved_40%_1/1 -> Data Type Conversion2/1, Enabled Subsystem1/Enable, Enabled Subsystem2/Enable, Enabled Subsystem3/Enable

== system HDVPSG_DelayComp_NewRef_RealDrop_case1/Subsystem6 ==
  vxr_HDV_first : Inport
  Dist_to_MP : Inport  Port=2
  Constant52 : Constant  Value=HDV_first_v0
  HDV_first : Subsystem
  Subsystem16 : Subsystem
  Subsystem17 : Subsystem
  Subsystem18 : Subsystem
  Subsystem7 : Subsystem
  vx_HDV_first : Outport
  HighMu : Outport  Port=2
  wires:
  Subsystem18/1(HDV_D) -> HDV_first/4(PID_D)
  Subsystem16/1(HDV_P) -> HDV_first/2(PID_P)
  vxr_HDV_first/1 -> HDV_first/1(vxr)
  Subsystem7/1(HDV_Mu) -> HDV_first/5(TRFC)
  Constant52/1 -> HDV_first/6(v_ini)
  Subsystem17/1(HDV_I) -> HDV_first/3(PID_I)
  HDV_first/1(vx) -> vx_HDV_first/1
  Dist_to_MP/1 -> Subsystem16/1(Dist_to_MP), Subsystem17/1(Dist_to_MP), Subsystem18/1(Dist_to_MP), Subsystem7/1(Dist_to_MP)
  Subsystem16/2(HighMu) -> HighMu/1

== system HDVPSG_DelayComp_NewRef_RealDrop_case1/Subsystem7 ==
  note: We assume you know if a packet is lost or not.
  Front_to_end : Inport
  v_Front : Inport  Port=2
  a_Front : Inport  Port=3
  Add : Sum
  Constant : Constant
  Data Type Conversion2 : DataTypeConversion
  Enabled Subsystem1 : Subsystem  TreatAsAtomicUnit=on
  Enabled Subsystem2 : Subsystem  TreatAsAtomicUnit=on
  Enabled Subsystem3 : Subsystem  TreatAsAtomicUnit=on
  Memory : Memory
  Mux : Mux  Inputs=2
  Mux1 : Mux  Inputs=2
  Mux2 : Mux  Inputs=2
  Recved_40%_3 : Lookup_n-D  NumberOfTableDimensions=1  BreakpointsForDimension1=1:3000  Table=Recved_40_3  InternalRulePriority=Speed  RndMeth=Simplest  InputSameDT=on
  Scope{,1..2,4} (4 alike) : Scope
  Front_to_end_PDR : Outport
  v_Front_PDR : Outport  Port=2
  a_Front_PDR : Outport  Port=3
  Recved : Outport  Port=4
  wires:
  Add/1 -> Memory/1
  Memory/1 -> Add/2, Recved_40%_3/1  "Index_Step"
  Enabled Subsystem1/1(Front_to_end_PDR) -> Mux/1, Front_to_end_PDR/1
  Enabled Subsystem3/1(a_Front_PDR) -> Mux2/1, a_Front_PDR/1
  a_Front/1 -> Mux2/2, Enabled Subsystem3/1(a_Front)
  Front_to_end/1 -> Mux/2, Enabled Subsystem1/1(Front_to_end)
  Mux/1 -> Scope/1
  Mux1/1 -> Scope1/1
  v_Front/1 -> Mux1/2, Enabled Subsystem2/1(v_Front)
  Enabled Subsystem2/1(v_Front_PDR) -> Mux1/1, v_Front_PDR/1
  Mux2/1 -> Scope2/1
  Data Type Conversion2/1 -> Recved/1, Scope4/1
  Constant/1 -> Add/1
  Recved_40%_3/1 -> Data Type Conversion2/1, Enabled Subsystem1/Enable, Enabled Subsystem2/Enable, Enabled Subsystem3/Enable

== system HDVPSG_DelayComp_NewRef_RealDrop_case1/Subsystem8 ==
  dis_to_MP : Inport
  Add5 : Sum
  Compare To Constant1 : simulink/Logic and Bit Operations/Compare To Constant  relop=<=  const=CtrlZone_Length  OutDataTypeStr=boolean
  Compare To Constant2 : simulink/Logic and Bit Operations/Compare To Constant  relop=>  const=0  OutDataTypeStr=boolean
  Data Type Conversion : DataTypeConversion
  Delay : Delay  DelayLength=1
  Ctrl_enabled : Outport
  Ctrl_enable_Index : Outport  Port=2
  wires:
  dis_to_MP/1 -> Compare To Constant1/1
  Compare To Constant1/1 -> Data Type Conversion/1
  Compare To Constant2/1 -> Ctrl_enabled/1
  Add5/1 -> Delay/1
  Delay/1 -> Compare To Constant2/1, Add5/2, Ctrl_enable_Index/1
  Data Type Conversion/1 -> Add5/1

== system HDVPSG_DelayComp_NewRef_RealDrop_case1/Subsystem9 ==
  dis_to_MP : Inport
  Add5 : Sum
  Compare To Constant1 : simulink/Logic and Bit Operations/Compare To Constant  relop=<=  const=CtrlZone_Length  OutDataTypeStr=boolean
  Compare To Constant2 : simulink/Logic and Bit Operations/Compare To Constant  relop=>  const=0  OutDataTypeStr=boolean
  Data Type Conversion : DataTypeConversion
  Delay : Delay  DelayLength=1
  Ctrl_enabled : Outport
  Ctrl_enable_Index : Outport  Port=2
  wires:
  Data Type Conversion/1 -> Add5/1
  Delay/1 -> Ctrl_enable_Index/1, Add5/2, Compare To Constant2/1
  Add5/1 -> Delay/1
  Compare To Constant2/1 -> Ctrl_enabled/1
  Compare To Constant1/1 -> Data Type Conversion/1
  dis_to_MP/1 -> Compare To Constant1/1

== system HDVPSG_DelayComp_NewRef_RealDrop_case1/leader_ulmpc_spd_ctrl ==
  note: Local (distributed) planning & control
      | based on the merging speed ref from RSU
  HDV_First_v : Inport
  HDV_First_v_dot_hat : Inport  Port=2
  spd_ini_ctzone : Inport  Port=3
  acc_ini_ctzone : Inport  Port=4
  Enable : EnablePort
  CVXGEN_Leader_ULMPC_Spd_Ctrl_ : S-Function  Description=Simulink:masks:SFunctionBuilder_MD  InitFcn=try, set_param(gcb,'FunctionName','CVXGEN_Leader_Spd_ULMPC'), end  FunctionName=CVXGEN_Leader_Spd_ULMPC  SFunctionModules=CVXGEN_Leader_Spd_ULMPC_wrapper solver util matrix_support ldl  SFunctionDeploymentMode=off  EnableBusSupport=off
      mask init: same as HDVPSG_DelayComp_NewRef_RealDrop_case1/HDV2_control_withPDR_compen/CVXGEN_Following_Car_Dist_Ctrl_NonSoft2
      settings: CopyFcn=set_param(gcbh,'LinkStatus','none')  PreSaveFcn=try, set_param(gcb,'FunctionName','CVXGEN_Leader_Spd_ULMPC'), end  OpenFcn=sfunctionwizard(gcbh)
      mask Display: plot(val(:,1),val(:,2)),disp(sys), port_label('input',1,'vmax'), port_label('input',2,'vmin'), port_label('input',3,'deltav_max'), port_label('input',4,'deltav_min'), port_label('input',5,'vcmd_max'), port_label('input',6,'vcmd_min'), port_label('input',7,'delta_vcmd_max'), port_label('input',8,'delta_vcmd_min'), port_label('input',9,'A'), port_label('input',10,'B'), port_label('input',11,'d_k'), port_label('input',12,'Q'), port_label('input',13,'R'), port_label('input',14,'v_ref'), port_label('input',15,'v_cmd_last'), port_label('input',16,'x_0'), port_label('output',1,'delta_v_cmd_opt'), port_label('output',2,'v_cmd_opt')
  Constant42 : Constant  Value=Q_Leader
  Constant43 : Constant  Value=R_Leader
  Constant44 : Constant
  Constant5 : Constant  Value=CtrlZone_Length
  Constant54 : Constant  Value=HDV_AMAX*T_ADE
  Constant55 : Constant  Value=HDV_AMIN*T_ADE
  Constant57 : Constant  Value=V_MAX
  Constant58 : Constant  Value=V_MIN
  Constant59 : Constant  Value=T_ADE
  Constant6 : Constant  Value=CtrlZone_Length
  Constant61 : Constant  Value=BETA_HDV_Leader
  Constant7 : Constant  Value=VR_MG_TCC
  Discrete-Time Integrator : DiscreteIntegrator  SampleTime=-1  ICPrevOutput=DiscIntNeverNeededParam  ICPrevScaledInput=DiscIntNeverNeededParam
  Fcn : Fcn  Expr=u(1)/((u(2)+u(3))/2)
  Gain : Gain  Gain=-1
  Gain1 : Gain  Gain=-1
  Memory2 : Memory  InitialCondition=HDV_first_v0
  Mux : Mux  Inputs=3
  Optimal_Control_Reference : MATLAB Function  TreatAsAtomicUnit=on
  Rate Transition{6,48..50,68,70..80} (16 alike) : RateTransition
  Scope1 : Scope
  Scope2 : Scope
  Scope3 : Scope
  Sys_Leader : MATLAB Function  TreatAsAtomicUnit=on
  delta_v_cmd_opt : Outport
  v_cmd_opt : Outport  Port=2
  vr : Outport  Port=3
  HDV1_t_all : Outport  Port=4
  HDV1_Run_t : Outport  Port=5
  opt_dist2MP : Outport  Port=6
  alpha_HDV1 : Outport  Port=7
  beta_HDV1 : Outport  Port=8
  c1_HDV1 : Outport  Port=9
  c2_HDV1 : Outport  Port=10
  c3_HDV1 : Outport  Port=11
  c4_HDV1 : Outport  Port=12
  wires:
  CVXGEN_Leader_ULMPC_Spd_Ctrl_/2 -> v_cmd_opt/1, Memory2/1  "v_cmd_opt"
  Sys_Leader/3(dk) -> Rate Transition48/1
  Rate Transition49/1 -> CVXGEN_Leader_ULMPC_Spd_Ctrl_/1
  Rate Transition50/1 -> CVXGEN_Leader_ULMPC_Spd_Ctrl_/2
  spd_ini_ctzone/1 -> Mux/2, Optimal_Control_Reference/2(v_ini)
  Constant61/1 -> Sys_Leader/2(beta)
  Sys_Leader/2(B) -> Rate Transition72/1
  Rate Transition77/1 -> CVXGEN_Leader_ULMPC_Spd_Ctrl_/7
  Constant59/1 -> Sys_Leader/1(Ts)
  Rate Transition75/1 -> CVXGEN_Leader_ULMPC_Spd_Ctrl_/13
  Constant55/1 -> Rate Transition70/1, Rate Transition78/1
  Constant54/1 -> Rate Transition68/1, Rate Transition77/1
  Rate Transition48/1 -> CVXGEN_Leader_ULMPC_Spd_Ctrl_/11
  Rate Transition72/1 -> CVXGEN_Leader_ULMPC_Spd_Ctrl_/10
  Rate Transition68/1 -> CVXGEN_Leader_ULMPC_Spd_Ctrl_/3
  Rate Transition70/1 -> CVXGEN_Leader_ULMPC_Spd_Ctrl_/4
  Constant58/1 -> Rate Transition50/1, Rate Transition76/1
  Rate Transition74/1 -> CVXGEN_Leader_ULMPC_Spd_Ctrl_/12
  Rate Transition76/1 -> CVXGEN_Leader_ULMPC_Spd_Ctrl_/6
  Constant57/1 -> Rate Transition49/1, Rate Transition73/1
  Constant42/1 -> Rate Transition74/1
  Rate Transition6/1 -> CVXGEN_Leader_ULMPC_Spd_Ctrl_/16
  Sys_Leader/1(A) -> Rate Transition71/1
  CVXGEN_Leader_ULMPC_Spd_Ctrl_/1 -> delta_v_cmd_opt/1
  Rate Transition71/1 -> CVXGEN_Leader_ULMPC_Spd_Ctrl_/9
  Rate Transition73/1 -> CVXGEN_Leader_ULMPC_Spd_Ctrl_/5
  Memory2/1 -> Rate Transition80/1
  Rate Transition80/1 -> CVXGEN_Leader_ULMPC_Spd_Ctrl_/15
  Rate Transition78/1 -> CVXGEN_Leader_ULMPC_Spd_Ctrl_/8
  Rate Transition79/1 -> CVXGEN_Leader_ULMPC_Spd_Ctrl_/14  "21"
  HDV_First_v/1 -> Rate Transition6/1
  Constant43/1 -> Rate Transition75/1
  Discrete-Time Integrator/1 -> HDV1_Run_t/1, Optimal_Control_Reference/6(t_aft_trigger)
  Constant44/1 -> Discrete-Time Integrator/1
  HDV_First_v_dot_hat/1 -> Sys_Leader/3(v_dot_hat)
  Constant6/1 -> Optimal_Control_Reference/1(L_ctz)
  acc_ini_ctzone/1 -> Optimal_Control_Reference/3(a_ini)
  Fcn/1 -> HDV1_t_all/1, Optimal_Control_Reference/5(T_rest_to_MP)
  Mux/1 -> Fcn/1
  Constant5/1 -> Mux/1
  Constant7/1 -> Optimal_Control_Reference/4(v_mp), Mux/3
  Optimal_Control_Reference/3(opt_acc) -> Scope1/1
  Optimal_Control_Reference/1(opt_pos) -> Gain/1
  Gain/1 -> opt_dist2MP/1
  Optimal_Control_Reference/2(opt_spd) -> vr/1
  Optimal_Control_Reference/5(opt_spd_vec) -> Rate Transition79/1, Scope2/1
  Optimal_Control_Reference/4(opt_pos_vec) -> Gain1/1
  Gain1/1 -> Scope3/1
  Optimal_Control_Reference/6(alpha) -> alpha_HDV1/1
  Optimal_Control_Reference/7(beta) -> beta_HDV1/1
  Optimal_Control_Reference/8(c_1) -> c1_HDV1/1
  Optimal_Control_Reference/9(c_2) -> c2_HDV1/1
  Optimal_Control_Reference/10(c_3) -> c3_HDV1/1
  Optimal_Control_Reference/11(c_4) -> c4_HDV1/1

== system HDVPSG_DelayComp_NewRef_RealDrop_case1/HDV2_control_withPDR_compen/Enabled and Triggered Subsystem ==
  delta_d_pre : Inport
  Enable : EnablePort
  delta_d_pre_freeze : Outport
  wires:
  delta_d_pre/1 -> delta_d_pre_freeze/1

== system HDVPSG_DelayComp_NewRef_RealDrop_case1/HDV2_control_withPDR_compen/Subsystem ==
  Recv : Inport
  Compare To Zero1 : simulink/Logic and Bit Operations/Compare To Zero  relop===  OutDataTypeStr=boolean
  Constant3 : Constant  Value=0
  Enabled and Triggered Subsystem1 : Subsystem  TreatAsAtomicUnit=on
  Switch : Switch  Criteria=u2 > Threshold
  Lost_Step : Outport
  wires:
  Compare To Zero1/1 -> Switch/2, Enabled and Triggered Subsystem1/Enable
  Enabled and Triggered Subsystem1/1(Lost_stop) -> Switch/1
  Constant3/1 -> Switch/3
  Recv/1 -> Compare To Zero1/1
  Switch/1 -> Lost_Step/1

== system HDVPSG_DelayComp_NewRef_RealDrop_case1/HDV2_control_withPDR_compen/Subsystem1 ==
  Lost_Step : Inport
  delta_d_pre_freeze_if_lost : Inport  Port=2
  delta_d_measure : Inport  Port=3
  Constant1 : Constant  Value=[1:1:Np_MPC+1]
  Lookup Table Dynamic : simulink/Lookup Tables/Lookup Table Dynamic  LookUpMeth=Interpolation-Extrapolation  OutDataType=fixdt('double')  OutScaling=[]  OutputDataTypeScalingMode=Specify via dialog  OutDataTypeStr=double  DoSatur=off
      settings: SourceProductName=Simulink
  MATLAB Function3 : MATLAB Function  TreatAsAtomicUnit=on
  Mux : Mux  Inputs=2
  Saturation : Saturate  UpperLimit=Np_MPC+1  LowerLimit=0
  Scope : Scope
  Switch : Switch  Criteria=u2 > Threshold  Threshold=Np_MPC+1
  delta_d_enhanced : Outport
  wires:
  delta_d_pre_freeze_if_lost/1 -> MATLAB Function3/2(delta_d_pre_freeze_if_lost), Lookup Table Dynamic/3
  delta_d_measure/1 -> MATLAB Function3/3(delta_d_measure)
  Constant1/1 -> Lookup Table Dynamic/2
  Lost_Step/1 -> Switch/2, Saturation/1, Lookup Table Dynamic/1
  Mux/1 -> Scope/1
  Switch/1 -> delta_d_enhanced/1
  Lookup Table Dynamic/1 -> Mux/1, Switch/1  "extrapolation_outside_Hp"
  MATLAB Function3/1(delta_d_MPC) -> Mux/2, Switch/3  "within Hp"
  Saturation/1 -> MATLAB Function3/1(Lost_Step)

== system HDVPSG_DelayComp_NewRef_RealDrop_case1/HDV2_control_withPDR_compen/Subsystem17 ==
  delta_dTCC : Inport
  T_end : Inport  Port=2
  veh0_dend_0 : Inport  Port=3
  veh2_dend_0 : Inport  Port=4
  veh0_v0 : Inport  Port=5
  veh2_v0 : Inport  Port=6
  Enable : EnablePort
  Add : Sum  Inputs=+-
  Add1 : Sum  Inputs=-+
  Poly_coefficient : MATLAB Function  TreatAsAtomicUnit=on
  a_0 : Outport
  a_1 : Outport  Port=2
  a_2 : Outport  Port=3
  a_3 : Outport  Port=4
  wires:
  Poly_coefficient/2(a_1) -> a_1/1
  Add/1 -> Poly_coefficient/1(delta_d0)
  Poly_coefficient/1(a_0) -> a_0/1
  T_end/1 -> Poly_coefficient/4(Tend)
  Add1/1 -> Poly_coefficient/3(delta_v0)  "delta_dr_dot"
  delta_dTCC/1 -> Poly_coefficient/2(delta_dTCC)
  Poly_coefficient/3(a_2) -> a_2/1
  Poly_coefficient/4(a_3) -> a_3/1
  veh0_dend_0/1 -> Add/2
  veh2_dend_0/1 -> Add/1
  veh2_v0/1 -> Add1/1
  veh0_v0/1 -> Add1/2

== system HDVPSG_DelayComp_NewRef_RealDrop_case1/HDV2_control_withPDR_compen/Subsystem18 ==
  a0 : Inport
  a1 : Inport  Port=2
  a2 : Inport  Port=3
  a3 : Inport  Port=4
  t_sumo : Inport  Port=5
  Ref : MATLAB Function  TreatAsAtomicUnit=on
  Ref_Pre_Vec : MATLAB Function  TreatAsAtomicUnit=on
  delta_dr : Outport
  delta_dr_dot : Outport  Port=2
  delta_dr_Pre_Vec : Outport  Port=3
  delta_dr_dot_Pre_Vec : Outport  Port=4
  wires:
  a2/1 -> Ref_Pre_Vec/3(a_2), Ref/3(a_2)
  Ref/2(delta_dr_dot) -> delta_dr_dot/1
  Ref/1(delta_dr) -> delta_dr/1
  t_sumo/1 -> Ref_Pre_Vec/5(t_sumo), Ref/5(t_sumo)
  a3/1 -> Ref_Pre_Vec/4(a_3), Ref/4(a_3)
  a1/1 -> Ref_Pre_Vec/2(a_1), Ref/2(a_1)
  a0/1 -> Ref_Pre_Vec/1(a_0), Ref/1(a_0)
  Ref_Pre_Vec/1(delta_dr_Pre_Vec) -> delta_dr_Pre_Vec/1
  Ref_Pre_Vec/2(delta_dr_dot_Pre_Vec) -> delta_dr_dot_Pre_Vec/1

== system HDVPSG_DelayComp_NewRef_RealDrop_case1/HDV2_control_withPDR_compen/Subsystem3 ==
  v_ego : Inport
  a_ego : Inport  Port=2
  t_all_leader : Inport  Port=3
  t_leader_has_run : Inport  Port=4
  Time_headway : Inport  Port=5
  t_PRE_has_run : Inport  Port=6
  Enable : EnablePort
  Add9 : Sum  Inputs=+-+
  v_ego_ini : Outport
  a_ego_ini : Outport  Port=2
  T_all_to_MP_ego : Outport  Port=3
  t_PRE_has_run_ini : Outport  Port=4
  wires:
  v_ego/1 -> v_ego_ini/1
  a_ego/1 -> a_ego_ini/1
  Add9/1 -> T_all_to_MP_ego/1
  t_leader_has_run/1 -> Add9/2
  Time_headway/1 -> Add9/3
  t_all_leader/1 -> Add9/1
  t_PRE_has_run/1 -> t_PRE_has_run_ini/1

== system HDVPSG_DelayComp_NewRef_RealDrop_case1/PSG1_control_withPDR_compen/Enabled and Triggered Subsystem ==
  delta_d_pre : Inport
  Enable : EnablePort
  delta_d_pre_freeze : Outport
  wires:
  delta_d_pre/1 -> delta_d_pre_freeze/1

== system HDVPSG_DelayComp_NewRef_RealDrop_case1/PSG1_control_withPDR_compen/Subsystem ==
  Recv : Inport
  Compare To Zero1 : simulink/Logic and Bit Operations/Compare To Zero  relop===  OutDataTypeStr=boolean
  Constant3 : Constant  Value=0
  Enabled and Triggered Subsystem1 : Subsystem  TreatAsAtomicUnit=on
  Switch : Switch  Criteria=u2 > Threshold
  Lost_Step : Outport
  wires:
  Switch/1 -> Lost_Step/1
  Recv/1 -> Compare To Zero1/1
  Constant3/1 -> Switch/3
  Enabled and Triggered Subsystem1/1(Lost_stop) -> Switch/1
  Compare To Zero1/1 -> Enabled and Triggered Subsystem1/Enable, Switch/2

== system HDVPSG_DelayComp_NewRef_RealDrop_case1/PSG1_control_withPDR_compen/Subsystem17 ==
  delta_dTCC : Inport
  T_end : Inport  Port=2
  veh0_dend_0 : Inport  Port=3
  veh2_dend_0 : Inport  Port=4
  veh0_v0 : Inport  Port=5
  veh2_v0 : Inport  Port=6
  Enable : EnablePort
  Add : Sum  Inputs=+-
  Add1 : Sum  Inputs=-+
  Poly_coefficient : MATLAB Function  TreatAsAtomicUnit=on
  a_0 : Outport
  a_1 : Outport  Port=2
  a_2 : Outport  Port=3
  a_3 : Outport  Port=4
  wires:
  veh0_v0/1 -> Add1/2
  veh2_v0/1 -> Add1/1
  veh2_dend_0/1 -> Add/1
  veh0_dend_0/1 -> Add/2
  Poly_coefficient/4(a_3) -> a_3/1
  Poly_coefficient/3(a_2) -> a_2/1
  delta_dTCC/1 -> Poly_coefficient/2(delta_dTCC)
  Add1/1 -> Poly_coefficient/3(delta_v0)  "delta_dr_dot"
  T_end/1 -> Poly_coefficient/4(Tend)
  Poly_coefficient/1(a_0) -> a_0/1
  Add/1 -> Poly_coefficient/1(delta_d0)
  Poly_coefficient/2(a_1) -> a_1/1

== system HDVPSG_DelayComp_NewRef_RealDrop_case1/PSG1_control_withPDR_compen/Subsystem18 ==
  a0 : Inport
  a1 : Inport  Port=2
  a2 : Inport  Port=3
  a3 : Inport  Port=4
  t_sumo : Inport  Port=5
  Ref : MATLAB Function  TreatAsAtomicUnit=on
  Ref_Pre_Vec : MATLAB Function  TreatAsAtomicUnit=on
  delta_dr : Outport
  delta_dr_dot : Outport  Port=2
  delta_dr_Pre_Vec : Outport  Port=3
  delta_dr_dot_Pre_Vec : Outport  Port=4
  wires:
  Ref_Pre_Vec/2(delta_dr_dot_Pre_Vec) -> delta_dr_dot_Pre_Vec/1
  Ref_Pre_Vec/1(delta_dr_Pre_Vec) -> delta_dr_Pre_Vec/1
  a0/1 -> Ref/1(a_0), Ref_Pre_Vec/1(a_0)
  a1/1 -> Ref/2(a_1), Ref_Pre_Vec/2(a_1)
  a3/1 -> Ref/4(a_3), Ref_Pre_Vec/4(a_3)
  t_sumo/1 -> Ref/5(t_sumo), Ref_Pre_Vec/5(t_sumo)
  Ref/1(delta_dr) -> delta_dr/1
  Ref/2(delta_dr_dot) -> delta_dr_dot/1
  a2/1 -> Ref/3(a_2), Ref_Pre_Vec/3(a_2)

== system HDVPSG_DelayComp_NewRef_RealDrop_case1/PSG1_control_withPDR_compen/Subsystem2 ==
  Lost_Step : Inport
  delta_d_pre_freeze_if_lost : Inport  Port=2
  delta_d_measure : Inport  Port=3
  Constant1 : Constant  Value=[1:1:Np_MPC+1]
  Lookup Table Dynamic : simulink/Lookup Tables/Lookup Table Dynamic  LookUpMeth=Interpolation-Extrapolation  OutDataType=fixdt('double')  OutScaling=[]  OutputDataTypeScalingMode=Specify via dialog  OutDataTypeStr=double  DoSatur=off
      settings: SourceProductName=Simulink
  MATLAB Function3 : MATLAB Function  TreatAsAtomicUnit=on
  Mux : Mux  Inputs=2
  Saturation : Saturate  UpperLimit=Np_MPC+1  LowerLimit=0
  Scope : Scope
  Switch : Switch  Criteria=u2 > Threshold  Threshold=Np_MPC+1
  delta_d_enhanced : Outport
  wires:
  delta_d_pre_freeze_if_lost/1 -> MATLAB Function3/2(delta_d_pre_freeze_if_lost), Lookup Table Dynamic/3
  delta_d_measure/1 -> MATLAB Function3/3(delta_d_measure)
  Constant1/1 -> Lookup Table Dynamic/2
  Lost_Step/1 -> Switch/2, Saturation/1, Lookup Table Dynamic/1
  Mux/1 -> Scope/1
  Switch/1 -> delta_d_enhanced/1
  Lookup Table Dynamic/1 -> Mux/1, Switch/1  "extrapolation_outside_Hp"
  MATLAB Function3/1(delta_d_MPC) -> Mux/2, Switch/3  "within Hp"
  Saturation/1 -> MATLAB Function3/1(Lost_Step)

== system HDVPSG_DelayComp_NewRef_RealDrop_case1/PSG1_control_withPDR_compen/Subsystem3 ==
  v_ego : Inport
  a_ego : Inport  Port=2
  t_all_leader : Inport  Port=3
  t_leader_has_run : Inport  Port=4
  Time_headway : Inport  Port=5
  t_PRE_has_run : Inport  Port=6
  Enable : EnablePort
  Add9 : Sum  Inputs=+-+
  v_ego_ini : Outport
  a_ego_ini : Outport  Port=2
  T_all_to_MP_ego : Outport  Port=3
  t_PRE_has_run_ini : Outport  Port=4
  wires:
  t_PRE_has_run/1 -> t_PRE_has_run_ini/1
  t_all_leader/1 -> Add9/1
  Time_headway/1 -> Add9/3
  t_leader_has_run/1 -> Add9/2
  Add9/1 -> T_all_to_MP_ego/1
  a_ego/1 -> a_ego_ini/1
  v_ego/1 -> v_ego_ini/1

== system HDVPSG_DelayComp_NewRef_RealDrop_case1/PSG2_control_withPDR_compen/Enabled and Triggered Subsystem ==
  delta_d_pre : Inport
  Enable : EnablePort
  delta_d_pre_freeze : Outport
  wires:
  delta_d_pre/1 -> delta_d_pre_freeze/1

== system HDVPSG_DelayComp_NewRef_RealDrop_case1/PSG2_control_withPDR_compen/Subsystem ==
  Recv : Inport
  Compare To Zero1 : simulink/Logic and Bit Operations/Compare To Zero  relop===  OutDataTypeStr=boolean
  Constant3 : Constant  Value=0
  Enabled and Triggered Subsystem1 : Subsystem  TreatAsAtomicUnit=on
  Switch : Switch  Criteria=u2 > Threshold
  Lost_Step : Outport
  wires:
  Compare To Zero1/1 -> Switch/2, Enabled and Triggered Subsystem1/Enable
  Enabled and Triggered Subsystem1/1(Lost_stop) -> Switch/1
  Constant3/1 -> Switch/3
  Recv/1 -> Compare To Zero1/1
  Switch/1 -> Lost_Step/1
